simulink model "motorcycle_pole_placement"  (R2021a)
settings: Solver=VariableStepAuto  StartTime=0.0  StopTime=10  RelTol=1e-3
values from neighbouring files (symbols this model uses):
  A = [0 0;1 0]    [pole_placement.m]
  B = [1; 0]    [pole_placement.m]
  C = [0 1]    [pole_placement.m]
  k = place(A,B,P)    [pole_placement.m]
undefined symbols (not defined in the file or in its folder): kr, L
settings Model: Creator=martina.elle  LastModifiedBy=francesco

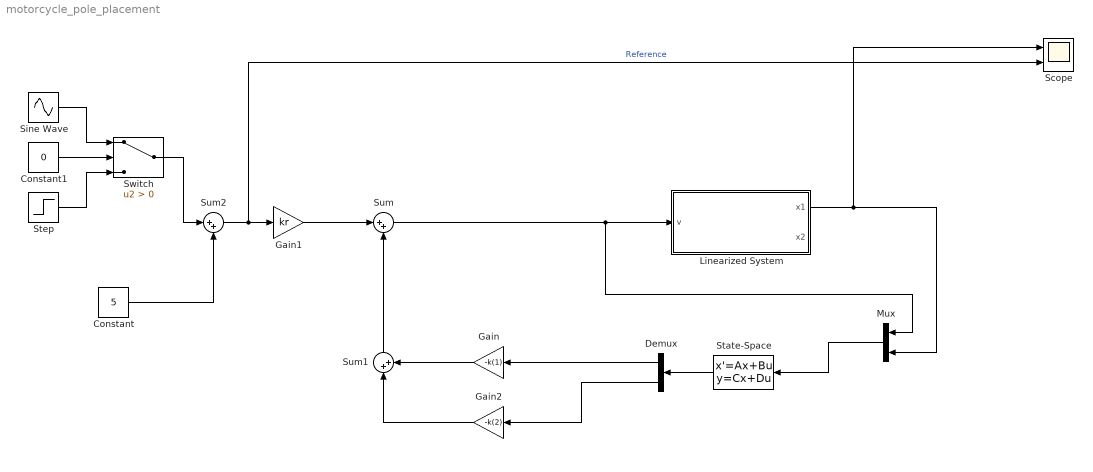
== system motorcycle_pole_placement ==
  Constant : Constant  Value=5
  Constant1 : Constant  Value=0
  Demux : Demux  Outputs=2
  Gain : Gain  Gain=-k(1)
  Gain1 : Gain  Gain=kr
  Gain2 : Gain  Gain=-k(2)
  Linearized System : Subsystem
  Mux : Mux  Inputs=2
  Scope : Scope  NumInputPorts=2
  Sine Wave : Sin  Amplitude=40  Frequency=0.1  SampleTime=0
  State-Space : StateSpace  A=A-L*C  B=[B L]  C=eye(2)  D=[0 0; 0 0]  InitialCondition=2  ParameterTunability=Unconstrained
  Step : Step  After=40  SampleTime=0
  Sum : Sum  Inputs=|++
  Sum1 : Sum  Inputs=|++
  Sum2 : Sum  Inputs=|++
  Switch : Switch  Criteria=u2 > Threshold
  wires:
  Gain1/1 -> Sum/1
  Mux/1 -> State-Space/1
  State-Space/1 -> Demux/1
  Demux/1 -> Gain/1
  Gain/1 -> Sum1/2
  Demux/2 -> Gain2/1
  Gain2/1 -> Sum1/1
  Sum1/1 -> Sum/2
  Switch/1 -> Sum2/1
  Constant/1 -> Sum2/2
  Constant1/1 -> Switch/2
  Sine Wave/1 -> Switch/1
  Step/1 -> Switch/3
  Sum2/1 -> Scope/2, Gain1/1  "Reference"
  Linearized System/1(x1) -> Mux/2, Scope/1
  Sum/1 -> Mux/1, Linearized System/1(v)

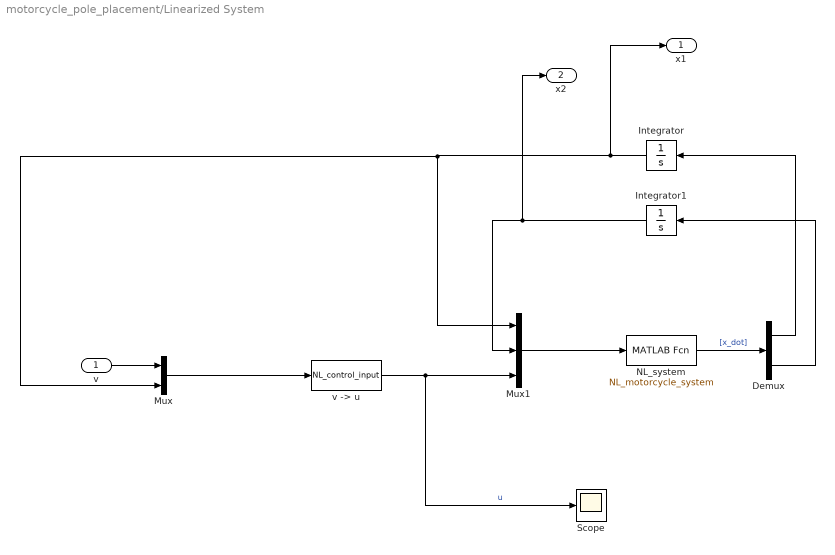
== system motorcycle_pole_placement/Linearized System ==
  v : Inport
  Demux : Demux  Outputs=2
  Integrator : Integrator  InitialCondition=10
  Integrator1 : Integrator  InitialCondition=10
  Mux : Mux  Inputs=2
  Mux1 : Mux  Inputs=3
  NL_system : MATLABFcn  MATLABFcn=NL_motorcycle_system  OutputDimensions=2
  Scope : Scope
  "v -> u" : MATLABFcn  MATLABFcn=NL_control_input  OutputDimensions=1
  x1 : Outport
  x2 : Outport  Port=2
  wires:
  NL_system/1 -> Demux/1  "[x_dot]"
  Integrator/1 -> x1/1, Mux/2, Mux1/1
  Integrator1/1 -> x2/1, Mux1/2
  Demux/2 -> Integrator1/1
  Demux/1 -> Integrator/1
  v/1 -> Mux/1
  Mux/1 -> "v -> u"/1
  Mux1/1 -> NL_system/1
  "v -> u"/1 -> Scope/1, Mux1/3  "u"
